simulink model "SystemModel"  (R2020b)
settings: Solver=VariableStepAuto  StartTime=0.0  StopTime=0.1  RelTol=1e-3
PostLoadFcn:
  | ModelInit
undefined symbols (not defined in the file): F_PWM
libraries: nesl_utility x25, fl_lib x24, ee_lib x22, powerlib_meascontrol x2
(part 1 of 2)
settings Model: Creator=on4ip  LastModifiedBy=on4ip
settings SolverCC: AutoInsertRateTranBlk=on
settings OptimizationCC: UseDivisionForNetSlopeComputation=on
settings ModelReferenceCC: EnableRefExpFcnMdlSchedulingChecks=off

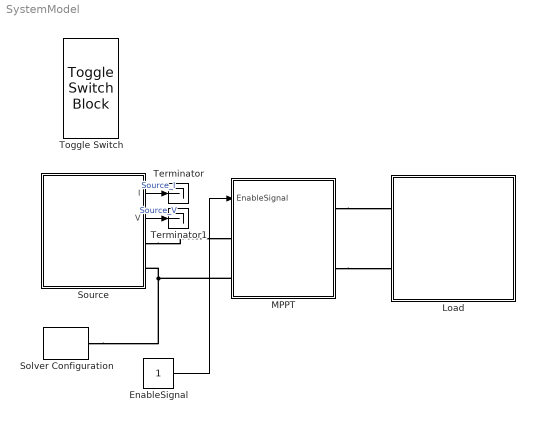
== system SystemModel ==
  EnableSignal : Constant
  Load : Subsystem
  MPPT : Subsystem
  Solver Configuration : nesl_utility/Solver Configuration  PhysicalDomain=network_engine_domain  SubClassName=solver  LeftPortType=input  RightPortType=generic  Tones=[]  Harmonics=[]  SimulateNoise=off  Profile=off  UseLocalSampling=off  EnableSwitchedLinearOptims=on  FrequencyDomain=off  UseCCode=off  RelTol=0.001  AbsTol=1e-06  MinStep=1e-09  ToWorkspace=off  RevertToSquareIcSolve=off  NumHomotopyIterations=100  PhasorMode=off  PhasorModeNumHarmonics=1  DoDC=on  ResidualTolerance=1e-09  UseLocalSolver=off  LocalSolverChoice=NE_BACKWARD_EULER_ADVANCER  LocalSolverSampleTime=1/10e6  DoFixedCost=off  MaxNonlinIter=3  MaxModeIter=2  ComputeImpulses=off  ImpulseIterations=2  LinearAlgebra=auto  EquationFormulation=NE_TIME_EF  DelaysMemoryBudget=1024  AutomaticFiltering=on  FilteringTimeConstant=0.001  PartitionStorageMethod=AS_NEEDED  PartitionMemoryBudget=1024  PartitionMethod=ROBUST
  Source : Subsystem  AncestorBlock=slexMaskingVariants_libraryblock/VariantSubsystem2  Variant=on  VariantControlMode=label  LabelModeActiveChoice=DCvariant  mask{VChoice=DC, Vnom=120}
      mask prompts: VChoice "Select a source variant"; Vnom "Nominal Voltage"
      mask init:
      | choice = get_param(gcb,'VChoice');
      | vssBlk = gcb;
      | oldVariant = get_param(gcb,'LabelModeActiveChoice');
      | if strcmp(choice,'DC')
      |     
      |     set_param(vssBlk, 'LabelModeActiveChoice', 'DCvariant');
      | else
      |     
      |     set_param(vssBlk, 'LabelModeActiveChoice', 'PVvariant');
      | end
      mask TypeOptions VChoice: DC | PV
      mask DialogControl DescGroupVar Prompt: Source Model Mask
      mask DialogControl DescTextVar Prompt: Выбор модели для источника питания
  Terminator : Terminator
  Terminator1 : Terminator
  Toggle Switch : ToggleSwitchBlock
      settings: Values={{'Off', 'On'}, [0 1]}
  wires:
  Source/1(I) -> Terminator/1  "Source_I"
  Source/2(V) -> Terminator1/1  "Source_V"
  EnableSignal/1 -> MPPT/1(EnableSignal)
  connections:
  Solver Configuration/RConn1 -- Source/RConn2 -- MPPT/LConn2
  Source/RConn1 -- MPPT/LConn1
  MPPT/RConn1 -- Load/LConn1
  MPPT/RConn2 -- Load/LConn2

== system SystemModel/Load ==
  Resistor : fl_lib/Electrical/Electrical Elements/Resistor  R=4 Ohm  i_specify=off  i_priority=None  i=0 A  i_nominal_specify=off  i_nominal_unit=A  i_nominal_value=1  v_specify=off  v_priority=None  v=0 V  v_nominal_specify=off  v_nominal_unit=V  v_nominal_value=1
  Load+ : PMIOPort  Side=Left
  Load- : PMIOPort  Port=2  Side=Left
  connections:
  Resistor/LConn1 -- Load+/RConn1
  Load-/RConn1 -- Resistor/RConn1

== system SystemModel/MPPT ==
  note: Для просмотра структуры конвертера
      | нажмите ЗДЕСЬ
  EnableSignal : Inport
  MCU : Subsystem
      settings: PortSchema="{\"entries\":[{\"content\":{\"sides\":[{\"content\":{\"connectorIds\":[\"Out1\"]},\"type\":\"ConnectorPlacement.EquallySpacedRectSide\",\"uuid\":\"95aacd01-5f53-4576-9898-5de1b84e2e57\"},{\"content\":{\"connectorIds\":[\"In1\"],\"side\":\"RIGHT\"},\"type\":\"ConnectorPlacement.EquallySpacedRectSide\",\"uuid\":\"70467306-ac55-4107-9f3e-d6d472329373\"},{\"content\":{\"connectorIds\":[],\"side\":\"TOP\"},\"type\":\"ConnectorPlacement.EquallySpacedRectSide\",\"uuid\":\"582591cf-2fae-45e2-b4f1-703e68dc17d8\"},{\"content\":{\"connectorIds\":[],\"side\":\"HIDDEN\"},\"type\":\"ConnectorPlacement.EquallySpacedRectSide\",\"uuid\":\"e5d6186a-71bc-43f6-a780-6a1a666a1cb3\"}]},\"type\":\"ConnectorPlacement.EquallySpacedConnector\",\"uuid\":\"3fd99db7-1fcf-4f0b-8db4-a60f3c66b2ee\"}],\"packageUris\":[\"http://schema.mathworks.com/mf0/Connector/R2020b\"],\"version\":\"1.0\"}"
  PhisicalModel : Subsystem
  IN+ : PMIOPort  Side=Left
  IN- : PMIOPort  Port=2  Side=Left
  Out+ : PMIOPort  Port=3  Side=Right
  Out- : PMIOPort  Port=4  Side=Right
  wires:
  MCU/1(Control_Signals) -> PhisicalModel/2(Control_Signals)
  PhisicalModel/1(Feedback_Signals) -> MCU/1(Feedback_Signals)
  EnableSignal/1 -> PhisicalModel/1(EnableSignal)
  connections:
  IN+/RConn1 -- PhisicalModel/LConn1
  IN-/RConn1 -- PhisicalModel/LConn2
  Out+/RConn1 -- PhisicalModel/RConn1
  Out-/RConn1 -- PhisicalModel/RConn2

== system SystemModel/Source ==
  note: 1) Add Subsystem or Model blocks as valid variant choices.
      | 2) You cannot connect blocks at this level. At simulation, connectivity is automatically
      | determined, based on the active variant and port name matching.
  DC source : Subsystem  VariantControl=DCvariant
  PV source : Subsystem  VariantControl=PVvariant
  + : PMIOPort  Side=Right
  - : PMIOPort  Port=2  Side=Right
  I : Outport  VectorParamsAs1DForOutWhenUnconnected=off
  V : Outport  Port=2  VectorParamsAs1DForOutWhenUnconnected=off

== system SystemModel/MPPT/MCU ==
  Feedback_Signals : Inport
  Bus Creator : BusCreator  Inputs=5
  Bus Selector : BusSelector  OutputSignals=PWM_ref,Ena,OPTO_1,OPTO_2,OPTO_3
  ControlMCU : ModelReference  ModelNameDialog=MpptControl.slx  SimulationMode=Normal  ScheduleRates=on  ModelReferenceVersion=1.23
      settings: PortSchema="{\"entries\":[{\"content\":{\"sides\":[{\"content\":{\"connectorIds\":[\"In2\",\"In1\"]},\"type\":\"ConnectorPlacement.EquallySpacedRectSide\",\"uuid\":\"62c77ea2-8a62-4ba9-937a-755ecaf63dee\"},{\"content\":{\"connectorIds\":[\"Out1\"],\"side\":\"RIGHT\"},\"type\":\"ConnectorPlacement.EquallySpacedRectSide\",\"uuid\":\"565939dd-5422-42ba-a796-bcc2d661967f\"},{\"content\":{\"connectorIds\":[],\"side\":\"TOP\"},\"type\":\"ConnectorPlacement.EquallySpacedRectSide\",\"uuid\":\"40f1e559-ba9a-42bc-8a75-57ac09117705\"},{\"content\":{\"connectorIds\":[],\"side\":\"HIDDEN\"},\"type\":\"ConnectorPlacement.EquallySpacedRectSide\",\"uuid\":\"e8af7b68-8515-405e-bf62-830d8685ff5a\"}]},\"type\":\"ConnectorPlacement.EquallySpacedConnector\",\"uuid\":\"8beb7fe5-f4a1-4e5e-a07e-3689976499a8\"}],\"packageUris\":[\"http://schema.mathworks.com/mf0/Connector/R2020b\"],\"version\":\"1.0\"}"
  MCU PWM : Subsystem  mask{Fpwm=F_PWM}
      mask prompts: Fpwm "PWM frequency"
  SignalPack : Subsystem
  Unit Delay : UnitDelay  SampleTime=-1  HasFrameUpgradeWarning=on
  Control_Signals : Outport
  wires:
  Bus Creator/1 -> Control_Signals/1
  Feedback_Signals/1 -> SignalPack/1(In1)
  MCU PWM/3(INB) -> Bus Creator/2  "INB"
  MCU PWM/2(INA) -> Bus Creator/1  "INA"
  Bus Selector/2 -> MCU PWM/2(Ena)  "<Ena>"
  Bus Selector/3 -> Bus Creator/3  "<OPTO_1>"
  Bus Selector/4 -> Bus Creator/4  "<OPTO_2>"
  Bus Selector/5 -> Bus Creator/5  "<OPTO_3>"
  ControlMCU/1 -> Unit Delay/1
  Unit Delay/1 -> Bus Selector/1
  SignalPack/1(FeedBack) -> ControlMCU/1
  Bus Selector/1 -> MCU PWM/1(Ref)  "<PWM_ref>"
  MCU PWM/1(ISR) -> ControlMCU/2

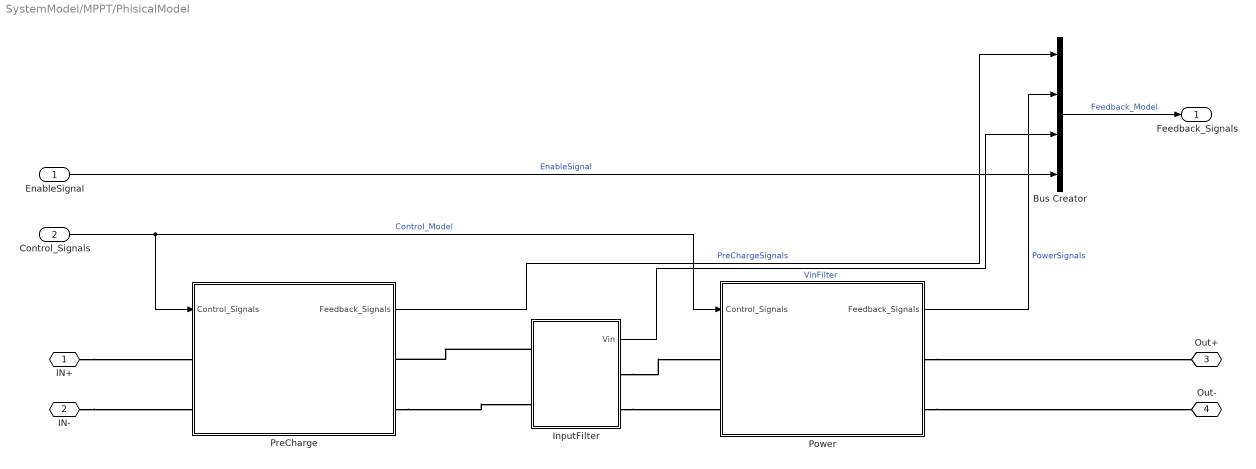
== system SystemModel/MPPT/PhisicalModel ==
  EnableSignal : Inport
  Control_Signals : Inport  Port=2
  Bus Creator : BusCreator  Inputs=4
  InputFilter : Subsystem  mask{Lf=20, Cf=11}
      mask prompts: Lf "Input filter Inductance,uH"; Cf "Input filter Capacitance,uF"
  Power : Subsystem  mask{Ls=200, Rs=30e-3, Cout=1000, Cf=2200, Lf=100}
      mask prompts: Ls "Inductor value,uH"; Rs "Inductor Resistance,Omh"; Cout "Out capacitor value,uF"; Cf "Filter capacitor value,uF"; Lf "Filter inductance value,uH"
  PreCharge : Subsystem
  IN+ : PMIOPort  Side=Left
  IN- : PMIOPort  Port=2  Side=Left
  Out+ : PMIOPort  Port=3  Side=Right
  Out- : PMIOPort  Port=4  Side=Right
  Feedback_Signals : Outport
  wires:
  Control_Signals/1 -> PreCharge/1(Control_Signals), Power/1(Control_Signals)  "Control_Model"
  Power/1(Feedback_Signals) -> Bus Creator/2  "PowerSignals"
  PreCharge/1(Feedback_Signals) -> Bus Creator/1  "PreChargeSignals"
  Bus Creator/1 -> Feedback_Signals/1  "Feedback_Model"
  InputFilter/1(Vin) -> Bus Creator/3  "VinFilter"
  EnableSignal/1 -> Bus Creator/4  "EnableSignal"
  connections:
  IN+/RConn1 -- PreCharge/LConn1
  IN-/RConn1 -- PreCharge/LConn2
  Power/RConn1 -- Out+/RConn1
  Power/RConn2 -- Out-/RConn1
  InputFilter/LConn1 -- PreCharge/RConn1
  PreCharge/RConn2 -- InputFilter/LConn2
  InputFilter/RConn1 -- Power/LConn1
  InputFilter/RConn2 -- Power/LConn2

== system SystemModel/Source/DC source ==
  Electrical Reference : fl_lib/Electrical/Electrical Elements/Electrical Reference
  Sensors : Subsystem
  Voltage Source : ee_lib/Sources/Voltage Source  dc_voltage=Vnom V  ac_voltage=0 V  ac_shift=0 rad  ac_frequency=60 Hz  noise_mode=0  PSD=0 V^2/Hz  repeatability=1  auto_seed=1503168829  user_seed=0  sample_time=1e-3 s  i_specify=off  i_priority=None  i=0 A  i_nominal_specify=off  i_nominal_unit=A  i_nominal_value=1  v_specify=off  v_priority=None  v=0 V  v_nominal_specify=off  v_nominal_unit=V  v_nominal_value=1
  + : PMIOPort  Side=Right
  - : PMIOPort  Port=2  Side=Right
  I : Outport  VectorParamsAs1DForOutWhenUnconnected=off
  V : Outport  Port=2  VectorParamsAs1DForOutWhenUnconnected=off
  wires:
  Sensors/1(I) -> I/1
  Sensors/2(V) -> V/1
  connections:
  Sensors/LConn1 -- Voltage Source/LConn1
  Voltage Source/RConn1 -- Electrical Reference/LConn1 -- Sensors/LConn2
  Sensors/RConn1 -- +/RConn1
  -/RConn1 -- Sensors/RConn2

== system SystemModel/Source/PV source ==
  Electrical Reference : fl_lib/Electrical/Electrical Elements/Electrical Reference
  Sensors : Subsystem
  Voltage Source : ee_lib/Sources/Voltage Source  dc_voltage=0 V  ac_voltage=0 V  ac_shift=0 rad  ac_frequency=60 Hz  noise_mode=0  PSD=0 V^2/Hz  repeatability=1  auto_seed=1582629291  user_seed=0  sample_time=1e-3 s  i_specify=off  i_priority=None  i=0 A  i_nominal_specify=off  i_nominal_unit=A  i_nominal_value=1  v_specify=off  v_priority=None  v=0 V  v_nominal_specify=off  v_nominal_unit=V  v_nominal_value=1
  + : PMIOPort  Side=Right
  - : PMIOPort  Port=2  Side=Right
  I : Outport  VectorParamsAs1DForOutWhenUnconnected=off
  V : Outport  Port=2  VectorParamsAs1DForOutWhenUnconnected=off
  wires:
  Sensors/1(I) -> I/1
  Sensors/2(V) -> V/1
  connections:
  Sensors/RConn1 -- +/RConn1
  Sensors/LConn1 -- Voltage Source/LConn1
  -/RConn1 -- Sensors/RConn2
  Voltage Source/RConn1 -- Electrical Reference/LConn1 -- Sensors/LConn2

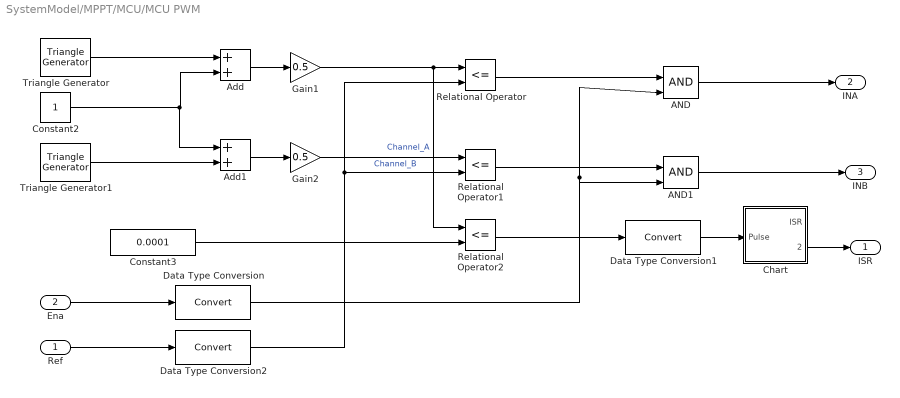
== system SystemModel/MPPT/MCU/MCU PWM ==
  Ref : Inport
  Ena : Inport  Port=2
  AND : Logic  IconShape=distinctive  AllPortsSameDT=off  OutDataTypeStr=boolean
  AND1 : Logic  IconShape=distinctive  AllPortsSameDT=off  OutDataTypeStr=boolean
  Add : Sum
  Add1 : Sum
  Chart : Stateflow chart  TreatAsAtomicUnit=on
  Constant2 : Constant
  Constant3 : Constant  Value=0.0001
  Data Type Conversion : DataTypeConversion
  Data Type Conversion1 : DataTypeConversion
  Data Type Conversion2 : DataTypeConversion
  Gain1 : Gain  Gain=0.5
  Gain2 : Gain  Gain=0.5
  Relational Operator : RelationalOperator  Operator=<=  OutDataTypeStr=boolean  ZeroCross=off  RndMeth=Simplest
  Relational Operator1 : RelationalOperator  Operator=<=  OutDataTypeStr=boolean  ZeroCross=off  RndMeth=Simplest
  Relational Operator2 : RelationalOperator  Operator=<=  OutDataTypeStr=boolean  RndMeth=Simplest
  Triangle Generator : powerlib_meascontrol/Pulse & Signal Generators/Triangle Generator  Freq=Fpwm  Phase=0  Ts=1/(Fpwm*100)
  Triangle Generator1 : powerlib_meascontrol/Pulse & Signal Generators/Triangle Generator  Freq=Fpwm  Phase=180  Ts=1/(Fpwm*100)
  ISR : Outport
  INA : Outport  Port=2
  INB : Outport  Port=3
  wires:
  Add/1 -> Gain1/1
  Relational Operator/1 -> AND/1
  Relational Operator1/1 -> AND1/1
  Ena/1 -> Data Type Conversion/1
  Ref/1 -> Data Type Conversion2/1
  Add1/1 -> Gain2/1
  Triangle Generator/1 -> Add/1
  Constant2/1 -> Add1/1, Add/2
  Triangle Generator1/1 -> Add1/2
  Gain1/1 -> Relational Operator2/1, Relational Operator/1  "Channel_A"
  Gain2/1 -> Relational Operator1/1  "Channel_B"
  Relational Operator2/1 -> Data Type Conversion1/1
  Constant3/1 -> Relational Operator2/2
  Data Type Conversion/1 -> AND/2, AND1/2
  Data Type Conversion2/1 -> Relational Operator/2, Relational Operator1/2
  AND/1 -> INA/1
  AND1/1 -> INB/1
  Data Type Conversion1/1 -> Chart/1(Pulse)
  Chart/2(ISR_event()) -> ISR/1

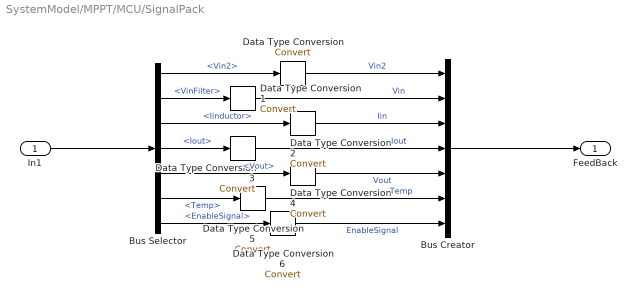
== system SystemModel/MPPT/MCU/SignalPack ==
  In1 : Inport
  Bus Creator : BusCreator  Inputs=7
  Bus Selector : BusSelector  OutputSignals=PreChargeSignals.Vin2,VinFilter,PowerSignals.Iinductor,PowerSignals.Iout,PowerSignals.Vout,PowerSignals.Temp,EnableSignal
  Data Type Conversion{,1..6} (7 alike) : DataTypeConversion
  FeedBack : Outport
  wires:
  Bus Selector/1 -> Data Type Conversion/1  "<Vin2>"
  Bus Selector/3 -> Data Type Conversion2/1  "<Iinductor>"
  Bus Selector/4 -> Data Type Conversion3/1  "<Iout>"
  Bus Selector/5 -> Data Type Conversion4/1  "<Vout>"
  Bus Selector/6 -> Data Type Conversion5/1  "<Temp>"
  Data Type Conversion/1 -> Bus Creator/1  "Vin2"
  Data Type Conversion1/1 -> Bus Creator/2  "Vin"
  Data Type Conversion2/1 -> Bus Creator/3  "Iin"
  Data Type Conversion3/1 -> Bus Creator/4  "Iout"
  Data Type Conversion4/1 -> Bus Creator/5  "Vout"
  Data Type Conversion5/1 -> Bus Creator/6  "Temp"
  In1/1 -> Bus Selector/1
  Bus Creator/1 -> FeedBack/1
  Bus Selector/2 -> Data Type Conversion1/1  "<VinFilter>"
  Bus Selector/7 -> Data Type Conversion6/1  "<EnableSignal>"
  Data Type Conversion6/1 -> Bus Creator/7  "EnableSignal"

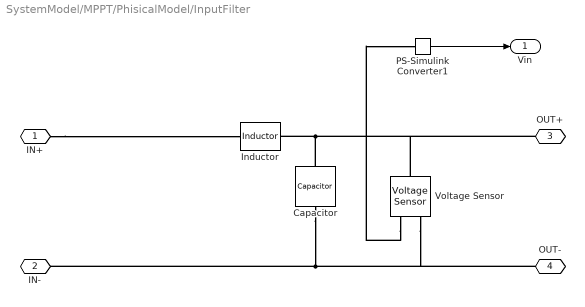
== system SystemModel/MPPT/PhisicalModel/InputFilter ==
  Capacitor : fl_lib/Electrical/Electrical Elements/Capacitor  c=Cf uF  r=1e-6 Ohm  g=0 1/Ohm  i_specify=off  i_priority=None  i=0 A  i_nominal_specify=off  i_nominal_unit=A  i_nominal_value=1  v_specify=off  v_priority=None  v=0 V  v_nominal_specify=off  v_nominal_unit=V  v_nominal_value=1  vc_specify=off  vc_priority=High  vc=0 V  vc_nominal_specify=off  vc_nominal_unit=V  vc_nominal_value=1
  Inductor : ee_lib/Passive/Inductor  l=Lf uH  L_tol=20  enable_L_tol=0  tol_distribution=1  nSigma=4  r=1e-3 Ohm  g=1e-9 1/Ohm  enable_operating_limits=0  operating_limit_action=2  max_working_current=1 A  power_rating=1 W  enable_faults=0  fault_action=1  lambdaPercent=50  k_faulted=0.9999  turnsShort=0  openCct=0  groundShort=0  groundShortG=0 1/Ohm  tau_fault=1e-3 s  enable_temporal_fault=0  t_fault=1 s  enable_behavioral_fault=0  max_permissible_voltage=100 V  n_fail_on_voltage=1  max_permissible_current=1 A  t_fail_on_current=1 s  i_L_specify=off  i_L_priority=High  i_L=0 A  i_L_nominal_specify=off  i_L_nominal_unit=A  i_L_nominal_value=1
  PS-Simulink Converter1 : nesl_utility/PS-Simulink Converter  PhysicalDomain=network_engine_domain  SubClassName=ps_output  LeftPortType=input  RightPortType=output  PseudoPeriodic=off  Frequencies=[]  Unit=inherit  AffineConversion=off
  Voltage Sensor : fl_lib/Electrical/Electrical Sensors/Voltage Sensor
  IN+ : PMIOPort  Side=Left
  IN- : PMIOPort  Port=2  Side=Left
  OUT+ : PMIOPort  Port=3  Side=Right
  OUT- : PMIOPort  Port=4  Side=Right
  Vin : Outport
  wires:
  PS-Simulink Converter1/1 -> Vin/1
  connections:
  IN+/RConn1 -- Inductor/LConn1
  Capacitor/LConn1 -- Voltage Sensor/LConn1 -- OUT+/RConn1 -- Inductor/RConn1
  Capacitor/RConn1 -- Voltage Sensor/RConn2 -- OUT-/RConn1 -- IN-/RConn1
  Voltage Sensor/RConn1 -- PS-Simulink Converter1/LConn1

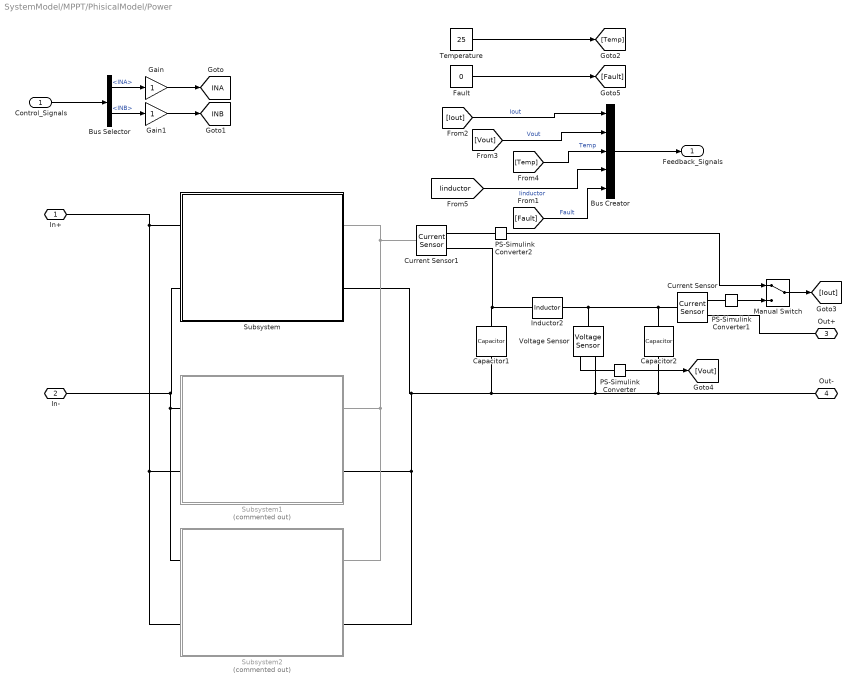
== system SystemModel/MPPT/PhisicalModel/Power ==
  Control_Signals : Inport
  Bus Creator : BusCreator  Inputs=5
  Bus Selector : BusSelector  OutputSignals=INA,INB
  Capacitor1 : fl_lib/Electrical/Electrical Elements/Capacitor  c=Cout uF  r=1e-6 Ohm  g=0 1/Ohm  i_specify=off  i_priority=None  i=0 A  i_nominal_specify=off  i_nominal_unit=A  i_nominal_value=1  v_specify=off  v_priority=None  v=0 V  v_nominal_specify=off  v_nominal_unit=V  v_nominal_value=1  vc_specify=off  vc_priority=High  vc=0 V  vc_nominal_specify=off  vc_nominal_unit=V  vc_nominal_value=1
  Capacitor2 : fl_lib/Electrical/Electrical Elements/Capacitor  c=Cf uF  r=1e-6 Ohm  g=0 1/Ohm  i_specify=off  i_priority=None  i=0 A  i_nominal_specify=off  i_nominal_unit=A  i_nominal_value=1  v_specify=off  v_priority=None  v=0 V  v_nominal_specify=off  v_nominal_unit=V  v_nominal_value=1  vc_specify=off  vc_priority=High  vc=0 V  vc_nominal_specify=off  vc_nominal_unit=V  vc_nominal_value=1
  Current Sensor : fl_lib/Electrical/Electrical Sensors/Current Sensor
  Current Sensor1 : fl_lib/Electrical/Electrical Sensors/Current Sensor
  Fault : Constant  Value=0  OutDataTypeStr=Inherit: Inherit via back propagation
  Gain : Gain  OutDataTypeStr=double
  Gain1 : Gain  OutDataTypeStr=double
  Inductor2 : ee_lib/Passive/Inductor  l=Lf nH  L_tol=20  enable_L_tol=0  tol_distribution=1  nSigma=4  r=0 Ohm  g=1e-9 1/Ohm  enable_operating_limits=0  operating_limit_action=2  max_working_current=1 A  power_rating=1 W  enable_faults=0  fault_action=1  lambdaPercent=50  k_faulted=0.9999  turnsShort=0  openCct=0  groundShort=0  groundShortG=0 1/Ohm  tau_fault=1e-3 s  enable_temporal_fault=0  t_fault=1 s  enable_behavioral_fault=0  max_permissible_voltage=100 V  n_fail_on_voltage=1  max_permissible_current=1 A  t_fail_on_current=1 s  i_L_specify=off  i_L_priority=High  i_L=0 A  i_L_nominal_specify=off  i_L_nominal_unit=A  i_L_nominal_value=1
  Manual Switch : ManualSwitch
  PS-Simulink Converter : nesl_utility/PS-Simulink Converter  PhysicalDomain=network_engine_domain  SubClassName=ps_output  LeftPortType=input  RightPortType=output  PseudoPeriodic=off  Frequencies=[]  Unit=inherit  AffineConversion=off
  PS-Simulink Converter1 : nesl_utility/PS-Simulink Converter  PhysicalDomain=network_engine_domain  SubClassName=ps_output  LeftPortType=input  RightPortType=output  PseudoPeriodic=off  Frequencies=[]  Unit=inherit  AffineConversion=off
  PS-Simulink Converter2 : nesl_utility/PS-Simulink Converter  PhysicalDomain=network_engine_domain  SubClassName=ps_output  LeftPortType=input  RightPortType=output  PseudoPeriodic=off  Frequencies=[]  Unit=inherit  AffineConversion=off
  Subsystem : Subsystem
  Subsystem1 : Subsystem  Commented=on
  Subsystem2 : Subsystem  Commented=on
  Temperature : Constant  Value=25  OutDataTypeStr=Inherit: Inherit via back propagation
  Voltage Sensor : fl_lib/Electrical/Electrical Sensors/Voltage Sensor
  In+ : PMIOPort  Side=Left
  In- : PMIOPort  Port=2  Side=Left
  Out+ : PMIOPort  Port=3  Side=Right
  Out- : PMIOPort  Port=4  Side=Right
  Feedback_Signals : Outport
  tag scope: INA=global, INB=global
  wires:
  Control_Signals/1 -> Bus Selector/1
  Bus Selector/1 -> Gain/1  "<INA>"
  Bus Selector/2 -> Gain1/1  "<INB>"
  Temperature/1 -> [Temp]
  PS-Simulink Converter/1 -> [Vout]
  Bus Creator/1 -> Feedback_Signals/1
  [Iout] -> Bus Creator/1  "Iout"
  [Temp] -> Bus Creator/3  "Temp"
  [Vout] -> Bus Creator/2  "Vout"
  Gain/1 -> [INA]
  Gain1/1 -> [INB]
  [Iinductor] -> Bus Creator/4  "Iinductor"
  PS-Simulink Converter2/1 -> Manual Switch/1
  PS-Simulink Converter1/1 -> Manual Switch/2
  Manual Switch/1 -> [Iout]
  Fault/1 -> [Fault]
  [Fault] -> Bus Creator/5  "Fault"
  connections:
  Subsystem/LConn2 -- Subsystem2/LConn1 -- Subsystem1/LConn1 -- In-/RConn1
  Inductor2/LConn1 -- Current Sensor1/RConn2 -- Capacitor1/LConn1
  Out+/RConn1 -- Current Sensor/RConn2
  Capacitor2/LConn1 -- Voltage Sensor/LConn1 -- Inductor2/RConn1 -- Current Sensor/LConn1
  PS-Simulink Converter/LConn1 -- Voltage Sensor/RConn1
  PS-Simulink Converter1/LConn1 -- Current Sensor/RConn1
  Subsystem/LConn1 -- Subsystem2/LConn2 -- Subsystem1/LConn2 -- In+/RConn1
  Voltage Sensor/RConn2 -- Subsystem2/RConn2 -- Subsystem1/RConn2 -- Subsystem/RConn2 -- Capacitor1/RConn1 -- Out-/RConn1 -- Capacitor2/RConn1
  Subsystem1/RConn1 -- Current Sensor1/LConn1 -- Subsystem/RConn1 -- Subsystem2/RConn1
  PS-Simulink Converter2/LConn1 -- Current Sensor1/RConn1

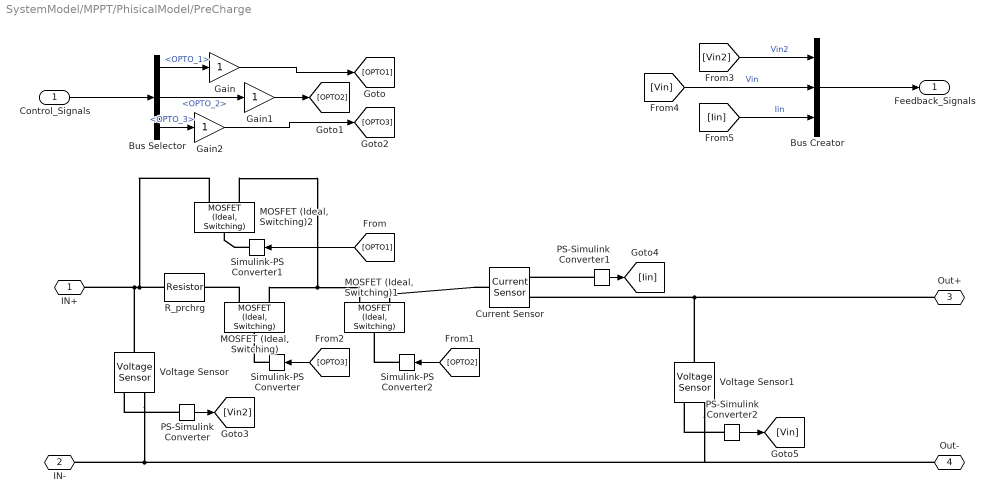
== system SystemModel/MPPT/PhisicalModel/PreCharge ==
  Control_Signals : Inport
  Bus Creator : BusCreator  Inputs=3
  Bus Selector : BusSelector  OutputSignals=OPTO_1,OPTO_2,OPTO_3
  Current Sensor : fl_lib/Electrical/Electrical Sensors/Current Sensor
  Gain : Gain  OutDataTypeStr=double
  Gain1 : Gain  OutDataTypeStr=double
  Gain2 : Gain  OutDataTypeStr=double
  "MOSFET (Ideal, Switching)" : ee_lib/Semiconductors & Converters/MOSFET (Ideal, Switching)  Rds=56e-3 Ohm  Goff=1e-6 1/Ohm  Vth=0.5 V  diode_param=2  diode_Vf=0.8 V  diode_Ron=0.001 Ohm  diode_Goff=1e-5 1/Ohm  diode_C=50e-9 F  diode_iRM=-235 A  diode_iF=300 A  diode_idot=-50 A/us  diode_trr_param=1  diode_trr_factor=3  diode_trr=15 us  diode_Qrr=1500 s*uA  thermal_loss_option=ee.enum.converters.thermalLossOption.constantvalues  Von_data=[0, 1.1, 1.3, 1.45, 1.75, 2.25, 2.7; 0, 1, 1.15, 1.35, 1.7, 2.35, 3] V  Eon_data=[0, .29, 1.43, 2.86, 5.71, 13.14, 22.86; 0, .57, 2.63, 5.14, 10.29, 20.57, 30.29] * 1e-3 J  Eoff_data=[0, .21, 1.07, 2.14, 4.29, 9.86, 17.14; 0, .43, 1.97, 3.86, 7.71, 15.43, 22.71] * 1e-3 J  Tj=[298.15, 398.15] K  Iout_data=[0, 10, 50, 100, 200, 400, 600] A  Eon_scalar=22.86e-3 J  Eoff_scalar=17.14e-3 J  Voff=300 V  Iout_scalar=600 A  diodeModelType=ee.enum.converters.diodeModelType.pwl  diode_IfMat=[.07, .12, .19, 1.75, 4.24, 7.32, 11.2; .16, .3, .72, 2.14, 4.02, 6.35, 9.12] A  diode_TjVec=[25, 125] degC  diode_VfVec=[.5, .7, .9, 1.3, 1.7, 2.1, 2.5] V  thermal_network_parameterization=ee.enum.thermalNetworkTopology.external  Rth=[.03, .2] K/W  Rth_Foster=[.03, .2] K/W  thermal_mass_parameterization=ee.enum.thermalNetwork.timeconstant  thermal_mass=[3, 25] J/K  thermal_mass_Foster=[33, 50] J/K  thermal_time_constant=[.1, 5] s  thermal_time_constant_Foster=[1, 10] s  thermal_mass_initial_temperatures=[25, 25] degC  junction_thermal_mass=0.1 J/K  Tau=1e-4 s  vT_specify=off  vT_priority=None  vT=0 V  vT_nominal_specify=off  vT_nominal_unit=V  vT_nominal_value=1  Qj_specify=off  Qj_priority=None  Qj=0 W  Qj_nominal_specify=off  Qj_nominal_unit=W  Qj_nominal_value=1  junction_temperature_specify=off  junction_temperature_priority=None  junction_temperature=25 degC  junction_temperature_nominal_specify=off  junction_temperature_nominal_unit=degC  junction_temperature_nominal_value=1
  "MOSFET (Ideal, Switching)1" : ee_lib/Semiconductors & Converters/MOSFET (Ideal, Switching)  Rds=56e-3 Ohm  Goff=1e-6 1/Ohm  Vth=0.5 V  diode_param=2  diode_Vf=0.8 V  diode_Ron=0.001 Ohm  diode_Goff=1e-5 1/Ohm  diode_C=50e-9 F  diode_iRM=-235 A  diode_iF=300 A  diode_idot=-50 A/us  diode_trr_param=1  diode_trr_factor=3  diode_trr=15 us  diode_Qrr=1500 s*uA  thermal_loss_option=ee.enum.converters.thermalLossOption.constantvalues  Von_data=[0, 1.1, 1.3, 1.45, 1.75, 2.25, 2.7; 0, 1, 1.15, 1.35, 1.7, 2.35, 3] V  Eon_data=[0, .29, 1.43, 2.86, 5.71, 13.14, 22.86; 0, .57, 2.63, 5.14, 10.29, 20.57, 30.29] * 1e-3 J  Eoff_data=[0, .21, 1.07, 2.14, 4.29, 9.86, 17.14; 0, .43, 1.97, 3.86, 7.71, 15.43, 22.71] * 1e-3 J  Tj=[298.15, 398.15] K  Iout_data=[0, 10, 50, 100, 200, 400, 600] A  Eon_scalar=22.86e-3 J  Eoff_scalar=17.14e-3 J  Voff=300 V  Iout_scalar=600 A  diodeModelType=ee.enum.converters.diodeModelType.pwl  diode_IfMat=[.07, .12, .19, 1.75, 4.24, 7.32, 11.2; .16, .3, .72, 2.14, 4.02, 6.35, 9.12] A  diode_TjVec=[25, 125] degC  diode_VfVec=[.5, .7, .9, 1.3, 1.7, 2.1, 2.5] V  thermal_network_parameterization=ee.enum.thermalNetworkTopology.external  Rth=[.03, .2] K/W  Rth_Foster=[.03, .2] K/W  thermal_mass_parameterization=ee.enum.thermalNetwork.timeconstant  thermal_mass=[3, 25] J/K  thermal_mass_Foster=[33, 50] J/K  thermal_time_constant=[.1, 5] s  thermal_time_constant_Foster=[1, 10] s  thermal_mass_initial_temperatures=[25, 25] degC  junction_thermal_mass=0.1 J/K  Tau=1e-4 s  vT_specify=off  vT_priority=None  vT=0 V  vT_nominal_specify=off  vT_nominal_unit=V  vT_nominal_value=1  Qj_specify=off  Qj_priority=None  Qj=0 W  Qj_nominal_specify=off  Qj_nominal_unit=W  Qj_nominal_value=1  junction_temperature_specify=off  junction_temperature_priority=None  junction_temperature=25 degC  junction_temperature_nominal_specify=off  junction_temperature_nominal_unit=degC  junction_temperature_nominal_value=1
  "MOSFET (Ideal, Switching)2" : ee_lib/Semiconductors & Converters/MOSFET (Ideal, Switching)  Rds=56e-3 Ohm  Goff=1e-6 1/Ohm  Vth=0.5 V  diode_param=2  diode_Vf=0.8 V  diode_Ron=0.001 Ohm  diode_Goff=1e-5 1/Ohm  diode_C=50e-9 F  diode_iRM=-235 A  diode_iF=300 A  diode_idot=-50 A/us  diode_trr_param=1  diode_trr_factor=3  diode_trr=15 us  diode_Qrr=1500 s*uA  thermal_loss_option=ee.enum.converters.thermalLossOption.constantvalues  Von_data=[0, 1.1, 1.3, 1.45, 1.75, 2.25, 2.7; 0, 1, 1.15, 1.35, 1.7, 2.35, 3] V  Eon_data=[0, .29, 1.43, 2.86, 5.71, 13.14, 22.86; 0, .57, 2.63, 5.14, 10.29, 20.57, 30.29] * 1e-3 J  Eoff_data=[0, .21, 1.07, 2.14, 4.29, 9.86, 17.14; 0, .43, 1.97, 3.86, 7.71, 15.43, 22.71] * 1e-3 J  Tj=[298.15, 398.15] K  Iout_data=[0, 10, 50, 100, 200, 400, 600] A  Eon_scalar=22.86e-3 J  Eoff_scalar=17.14e-3 J  Voff=300 V  Iout_scalar=600 A  diodeModelType=ee.enum.converters.diodeModelType.pwl  diode_IfMat=[.07, .12, .19, 1.75, 4.24, 7.32, 11.2; .16, .3, .72, 2.14, 4.02, 6.35, 9.12] A  diode_TjVec=[25, 125] degC  diode_VfVec=[.5, .7, .9, 1.3, 1.7, 2.1, 2.5] V  thermal_network_parameterization=ee.enum.thermalNetworkTopology.external  Rth=[.03, .2] K/W  Rth_Foster=[.03, .2] K/W  thermal_mass_parameterization=ee.enum.thermalNetwork.timeconstant  thermal_mass=[3, 25] J/K  thermal_mass_Foster=[33, 50] J/K  thermal_time_constant=[.1, 5] s  thermal_time_constant_Foster=[1, 10] s  thermal_mass_initial_temperatures=[25, 25] degC  junction_thermal_mass=0.1 J/K  Tau=1e-4 s  vT_specify=off  vT_priority=None  vT=0 V  vT_nominal_specify=off  vT_nominal_unit=V  vT_nominal_value=1  Qj_specify=off  Qj_priority=None  Qj=0 W  Qj_nominal_specify=off  Qj_nominal_unit=W  Qj_nominal_value=1  junction_temperature_specify=off  junction_temperature_priority=None  junction_temperature=25 degC  junction_temperature_nominal_specify=off  junction_temperature_nominal_unit=degC  junction_temperature_nominal_value=1
  PS-Simulink Converter : nesl_utility/PS-Simulink Converter  PhysicalDomain=network_engine_domain  SubClassName=ps_output  LeftPortType=input  RightPortType=output  PseudoPeriodic=off  Frequencies=[]  Unit=inherit  AffineConversion=off
  PS-Simulink Converter1 : nesl_utility/PS-Simulink Converter  PhysicalDomain=network_engine_domain  SubClassName=ps_output  LeftPortType=input  RightPortType=output  PseudoPeriodic=off  Frequencies=[]  Unit=inherit  AffineConversion=off
  PS-Simulink Converter2 : nesl_utility/PS-Simulink Converter  PhysicalDomain=network_engine_domain  SubClassName=ps_output  LeftPortType=input  RightPortType=output  PseudoPeriodic=off  Frequencies=[]  Unit=inherit  AffineConversion=off
  R_prchrg : fl_lib/Electrical/Electrical Elements/Resistor  R=100 Ohm  i_specify=off  i_priority=None  i=0 A  i_nominal_specify=off  i_nominal_unit=A  i_nominal_value=1  v_specify=off  v_priority=None  v=0 V  v_nominal_specify=off  v_nominal_unit=V  v_nominal_value=1
  Simulink-PS Converter : nesl_utility/Simulink-PS Converter  PhysicalDomain=network_engine_domain  SubClassName=ps_input  LeftPortType=input  RightPortType=output  PseudoPeriodic=off  Frequencies=[]  NoiseDistribution=none  NoiseParameters=[]  Unit=1  AffineConversion=off  FilteringAndDerivatives=provide  SimscapeFilterOrder=1  InputFilterTimeConstant=0.001  UdotUserProvided=0
  Simulink-PS Converter1 : nesl_utility/Simulink-PS Converter  PhysicalDomain=network_engine_domain  SubClassName=ps_input  LeftPortType=input  RightPortType=output  PseudoPeriodic=off  Frequencies=[]  NoiseDistribution=none  NoiseParameters=[]  Unit=1  AffineConversion=off  FilteringAndDerivatives=provide  SimscapeFilterOrder=1  InputFilterTimeConstant=0.001  UdotUserProvided=0
  Simulink-PS Converter2 : nesl_utility/Simulink-PS Converter  PhysicalDomain=network_engine_domain  SubClassName=ps_input  LeftPortType=input  RightPortType=output  PseudoPeriodic=off  Frequencies=[]  NoiseDistribution=none  NoiseParameters=[]  Unit=1  AffineConversion=off  FilteringAndDerivatives=provide  SimscapeFilterOrder=1  InputFilterTimeConstant=0.001  UdotUserProvided=0
  Voltage Sensor : fl_lib/Electrical/Electrical Sensors/Voltage Sensor
  Voltage Sensor1 : fl_lib/Electrical/Electrical Sensors/Voltage Sensor
  IN+ : PMIOPort  Side=Left
  IN- : PMIOPort  Port=2  Side=Left
  Out+ : PMIOPort  Port=3  Side=Right
  Out- : PMIOPort  Port=4  Side=Right
  Feedback_Signals : Outport
  wires:
  PS-Simulink Converter1/1 -> [Iin]
  Control_Signals/1 -> Bus Selector/1
  Bus Selector/1 -> Gain/1  "<OPTO_1>"
  Bus Selector/2 -> Gain1/1  "<OPTO_2>"
  Bus Selector/3 -> Gain2/1  "<OPTO_3>"
  [OPTO1] -> Simulink-PS Converter1/1
  [OPTO2] -> Simulink-PS Converter2/1
  [OPTO3] -> Simulink-PS Converter/1
  PS-Simulink Converter/1 -> [Vin2]
  PS-Simulink Converter2/1 -> [Vin]
  Bus Creator/1 -> Feedback_Signals/1
  [Vin2] -> Bus Creator/1  "Vin2"
  [Vin] -> Bus Creator/2  "Vin"
  [Iin] -> Bus Creator/3  "Iin"
  Gain/1 -> [OPTO1]
  Gain1/1 -> [OPTO2]
  Gain2/1 -> [OPTO3]
  connections:
  "MOSFET (Ideal, Switching)"/RConn2 -- "MOSFET (Ideal, Switching)2"/RConn2 -- "MOSFET (Ideal, Switching)1"/RConn2
  "MOSFET (Ideal, Switching)2"/RConn1 -- R_prchrg/LConn1 -- Voltage Sensor/LConn1 -- IN+/RConn1
  "MOSFET (Ideal, Switching)"/RConn1 -- R_prchrg/RConn1
  Voltage Sensor/RConn2 -- Out-/RConn1 -- Voltage Sensor1/RConn2 -- IN-/RConn1
  Current Sensor/LConn1 -- "MOSFET (Ideal, Switching)1"/RConn1
  Voltage Sensor1/LConn1 -- Out+/RConn1 -- Current Sensor/RConn2
  Simulink-PS Converter/RConn1 -- "MOSFET (Ideal, Switching)"/LConn1
  Simulink-PS Converter1/RConn1 -- "MOSFET (Ideal, Switching)2"/LConn1
  Simulink-PS Converter2/RConn1 -- "MOSFET (Ideal, Switching)1"/LConn1
  PS-Simulink Converter/LConn1 -- Voltage Sensor/RConn1
  PS-Simulink Converter1/LConn1 -- Current Sensor/RConn1
  PS-Simulink Converter2/LConn1 -- Voltage Sensor1/RConn1

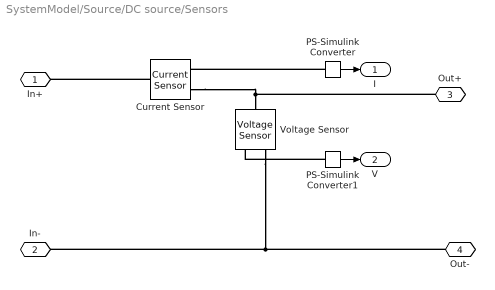
== system SystemModel/Source/DC source/Sensors ==
  Current Sensor : fl_lib/Electrical/Electrical Sensors/Current Sensor
  PS-Simulink Converter : nesl_utility/PS-Simulink Converter  PhysicalDomain=network_engine_domain  SubClassName=ps_output  LeftPortType=input  RightPortType=output  PseudoPeriodic=off  Frequencies=[]  Unit=inherit  AffineConversion=off
  PS-Simulink Converter1 : nesl_utility/PS-Simulink Converter  PhysicalDomain=network_engine_domain  SubClassName=ps_output  LeftPortType=input  RightPortType=output  PseudoPeriodic=off  Frequencies=[]  Unit=inherit  AffineConversion=off
  Voltage Sensor : fl_lib/Electrical/Electrical Sensors/Voltage Sensor
  In+ : PMIOPort  Side=Left
  In- : PMIOPort  Port=2  Side=Left
  Out+ : PMIOPort  Port=3  Side=Right
  Out- : PMIOPort  Port=4  Side=Right
  I : Outport
  V : Outport  Port=2
  wires:
  PS-Simulink Converter/1 -> I/1
  PS-Simulink Converter1/1 -> V/1
  connections:
  Current Sensor/RConn2 -- Out+/RConn1 -- Voltage Sensor/LConn1
  PS-Simulink Converter/LConn1 -- Current Sensor/RConn1
  Current Sensor/LConn1 -- In+/RConn1
  PS-Simulink Converter1/LConn1 -- Voltage Sensor/RConn1
  Out-/RConn1 -- In-/RConn1 -- Voltage Sensor/RConn2

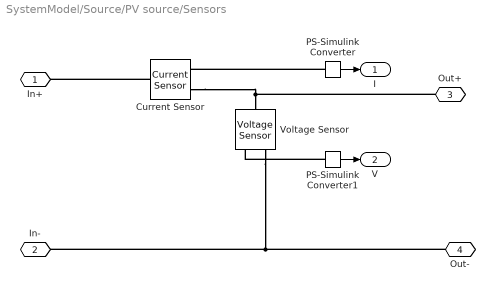
== system SystemModel/Source/PV source/Sensors ==
  Current Sensor : fl_lib/Electrical/Electrical Sensors/Current Sensor
  PS-Simulink Converter : nesl_utility/PS-Simulink Converter  PhysicalDomain=network_engine_domain  SubClassName=ps_output  LeftPortType=input  RightPortType=output  PseudoPeriodic=off  Frequencies=[]  Unit=inherit  AffineConversion=off
  PS-Simulink Converter1 : nesl_utility/PS-Simulink Converter  PhysicalDomain=network_engine_domain  SubClassName=ps_output  LeftPortType=input  RightPortType=output  PseudoPeriodic=off  Frequencies=[]  Unit=inherit  AffineConversion=off
  Voltage Sensor : fl_lib/Electrical/Electrical Sensors/Voltage Sensor
  In+ : PMIOPort  Side=Left
  In- : PMIOPort  Port=2  Side=Left
  Out+ : PMIOPort  Port=3  Side=Right
  Out- : PMIOPort  Port=4  Side=Right
  I : Outport
  V : Outport  Port=2
  wires:
  PS-Simulink Converter/1 -> I/1
  PS-Simulink Converter1/1 -> V/1
  connections:
  Voltage Sensor/LConn1 -- Current Sensor/RConn2 -- Out+/RConn1
  PS-Simulink Converter/LConn1 -- Current Sensor/RConn1
  Current Sensor/LConn1 -- In+/RConn1
  PS-Simulink Converter1/LConn1 -- Voltage Sensor/RConn1
  Voltage Sensor/RConn2 -- Out-/RConn1 -- In-/RConn1

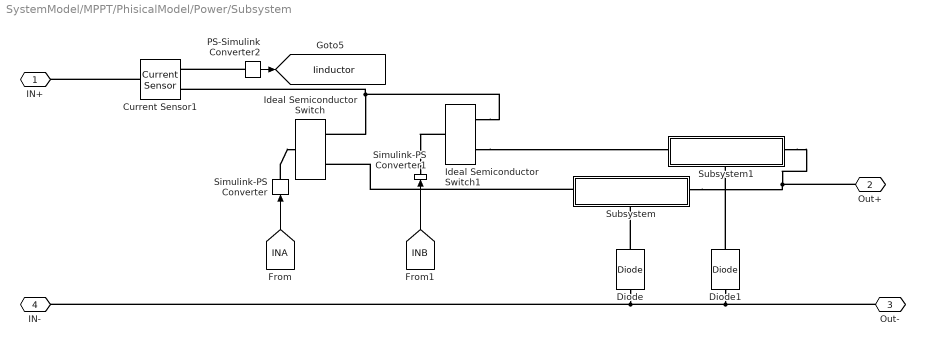
== system SystemModel/MPPT/PhisicalModel/Power/Subsystem ==
  Current Sensor1 : fl_lib/Electrical/Electrical Sensors/Current Sensor
  Diode : ee_lib/Semiconductors & Converters/Diode  ModelType=ee.enum.diode.modelType.pwl  IfMat=[.07, .12, .19, 1.75, 4.24, 7.32, 11.2; .16, .3, .72, 2.14, 4.02, 6.35, 9.12] A  TjVec=[25, 125] degC  VfVec=[.5, .7, .9, 1.3, 1.7, 2.1, 2.5] V  Vf=0.6 V  Ron=0.003 Ohm  Goff=1e-8 S  prmExp=ee.enum.diode.expParam.useTwo  I12=[.0137, .545] A  V12=[.6, .7] V  IS=1e-12 A  ec=1  I1=0.0137 A  V1=0.6 V  RS=0 Ohm  Tmeas=25 degC  N_series=1  N_parallel=1  Rz=0.3 Ohm  BV=inf V  C_param=ee.enum.diode.capParam.fixed  CJ=36 pF  CJ0=5 pF  VJ=1 V  Mgrad=0.5  Vvec=[.1, 10, 100] V  Cvec=[3.5, 1, .4] pF  FC=0.5  Q_param=ee.enum.diode.recoveryParam.off  iRM=-7.15 A  iF=4 A  didt=-750 A/us  trr_factor=3  trr=115 ns  Qrr=1500 s*uA  TT=50 ns  tau=100 ns  T_param=ee.enum.diode.temperatureParam.off  IS_T2=1.25e-7 A  I1_T2=0.245 A  V1_T2=0.5 V  Tmeas2=125 degC  EG_param=ee.enum.diode.egapParam.material_si  EG=1.11 eV  XTI_param=ee.enum.diode.xtiParam.pn  XTI=3  dBVdT=0 V/K  Tdevice=25 degC  i_specify=off  i_priority=None  i=0 A  i_nominal_specify=off  i_nominal_unit=A  i_nominal_value=1  v_specify=off  v_priority=None  v=0 V  v_nominal_specify=off  v_nominal_unit=V  v_nominal_value=1  i_capacitor_specify=off  i_capacitor_priority=None  i_capacitor=0 A  i_capacitor_nominal_specify=off  i_capacitor_nominal_unit=A  i_capacitor_nominal_value=1  v_capacitor_specify=off  v_capacitor_priority=None  v_capacitor=0 V  v_capacitor_nominal_specify=off  v_capacitor_nominal_unit=V  v_capacitor_nominal_value=1  power_dissipated_specify=off  power_dissipated_priority=None  power_dissipated=0 W  power_dissipated_nominal_specify=off  power_dissipated_nominal_unit=W  power_dissipated_nominal_value=1  thermal_network_parameterization=ee.enum.thermalNetworkTopology.cauer  Rth=[0, 10] K/W  Rth_Foster=[4, 6] K/W  thermal_mass_parameterization=ee.enum.thermalNetwork.timeconstant  thermal_mass=[0, 1] J/K  thermal_mass_Foster=[1.5, 3] J/K  thermal_time_constant=[0, 10] s  thermal_time_constant_Foster=[6, 18] s  thermal_mass_initial_temperatures=[25, 25] degC
  Diode1 : ee_lib/Semiconductors & Converters/Diode  ModelType=ee.enum.diode.modelType.pwl  IfMat=[.07, .12, .19, 1.75, 4.24, 7.32, 11.2; .16, .3, .72, 2.14, 4.02, 6.35, 9.12] A  TjVec=[25, 125] degC  VfVec=[.5, .7, .9, 1.3, 1.7, 2.1, 2.5] V  Vf=0.6 V  Ron=0.003 Ohm  Goff=1e-8 S  prmExp=ee.enum.diode.expParam.useTwo  I12=[.0137, .545] A  V12=[.6, .7] V  IS=1e-12 A  ec=1  I1=0.0137 A  V1=0.6 V  RS=0 Ohm  Tmeas=25 degC  N_series=1  N_parallel=1  Rz=0.3 Ohm  BV=inf V  C_param=ee.enum.diode.capParam.fixed  CJ=36 pF  CJ0=5 pF  VJ=1 V  Mgrad=0.5  Vvec=[.1, 10, 100] V  Cvec=[3.5, 1, .4] pF  FC=0.5  Q_param=ee.enum.diode.recoveryParam.off  iRM=-7.15 A  iF=4 A  didt=-750 A/us  trr_factor=3  trr=115 ns  Qrr=1500 s*uA  TT=50 ns  tau=100 ns  T_param=ee.enum.diode.temperatureParam.off  IS_T2=1.25e-7 A  I1_T2=0.245 A  V1_T2=0.5 V  Tmeas2=125 degC  EG_param=ee.enum.diode.egapParam.material_si  EG=1.11 eV  XTI_param=ee.enum.diode.xtiParam.pn  XTI=3  dBVdT=0 V/K  Tdevice=25 degC  i_specify=off  i_priority=None  i=0 A  i_nominal_specify=off  i_nominal_unit=A  i_nominal_value=1  v_specify=off  v_priority=None  v=0 V  v_nominal_specify=off  v_nominal_unit=V  v_nominal_value=1  i_capacitor_specify=off  i_capacitor_priority=None  i_capacitor=0 A  i_capacitor_nominal_specify=off  i_capacitor_nominal_unit=A  i_capacitor_nominal_value=1  v_capacitor_specify=off  v_capacitor_priority=None  v_capacitor=0 V  v_capacitor_nominal_specify=off  v_capacitor_nominal_unit=V  v_capacitor_nominal_value=1  power_dissipated_specify=off  power_dissipated_priority=None  power_dissipated=0 W  power_dissipated_nominal_specify=off  power_dissipated_nominal_unit=W  power_dissipated_nominal_value=1  thermal_network_parameterization=ee.enum.thermalNetworkTopology.cauer  Rth=[0, 10] K/W  Rth_Foster=[4, 6] K/W  thermal_mass_parameterization=ee.enum.thermalNetwork.timeconstant  thermal_mass=[0, 1] J/K  thermal_mass_Foster=[1.5, 3] J/K  thermal_time_constant=[0, 10] s  thermal_time_constant_Foster=[6, 18] s  thermal_mass_initial_temperatures=[25, 25] degC
  Ideal Semiconductor Switch : ee_lib/Semiconductors & Converters/Ideal Semiconductor Switch  Ron=0.001 Ohm  Goff=1e-6 1/Ohm  Vth=0.5 V  diode_param=2  diode_Vf=0.8 V  diode_Ron=0.001 Ohm  diode_Goff=1e-5 1/Ohm  diode_C=50e-9 F  diode_iRM=-235 A  diode_iF=300 A  diode_idot=-50 A/us  diode_trr_param=1  diode_trr_factor=3  diode_trr=15 us  diode_Qrr=1500 s*uA
      settings: SourceProductBaseCode=PS
  Ideal Semiconductor Switch1 : ee_lib/Semiconductors & Converters/Ideal Semiconductor Switch  Ron=0.001 Ohm  Goff=1e-6 1/Ohm  Vth=0.5 V  diode_param=2  diode_Vf=0.8 V  diode_Ron=0.001 Ohm  diode_Goff=1e-5 1/Ohm  diode_C=50e-9 F  diode_iRM=-235 A  diode_iF=300 A  diode_idot=-50 A/us  diode_trr_param=1  diode_trr_factor=3  diode_trr=15 us  diode_Qrr=1500 s*uA
      settings: SourceProductBaseCode=PS
  PS-Simulink Converter2 : nesl_utility/PS-Simulink Converter  PhysicalDomain=network_engine_domain  SubClassName=ps_output  LeftPortType=input  RightPortType=output  PseudoPeriodic=off  Frequencies=[]  Unit=inherit  AffineConversion=off
  Simulink-PS Converter : nesl_utility/Simulink-PS Converter  PhysicalDomain=network_engine_domain  SubClassName=ps_input  LeftPortType=input  RightPortType=output  PseudoPeriodic=off  Frequencies=[]  NoiseDistribution=none  NoiseParameters=[]  Unit=1  AffineConversion=off  FilteringAndDerivatives=provide  SimscapeFilterOrder=1  InputFilterTimeConstant=0.001  UdotUserProvided=0
  Simulink-PS Converter1 : nesl_utility/Simulink-PS Converter  PhysicalDomain=network_engine_domain  SubClassName=ps_input  LeftPortType=input  RightPortType=output  PseudoPeriodic=off  Frequencies=[]  NoiseDistribution=none  NoiseParameters=[]  Unit=1  AffineConversion=off  FilteringAndDerivatives=provide  SimscapeFilterOrder=1  InputFilterTimeConstant=0.001  UdotUserProvided=0
  Subsystem : Subsystem
      settings: PortSchema="{\"entries\":[{\"content\":{\"sides\":[{\"content\":{\"connectorIds\":[\"LConn1\"]},\"type\":\"ConnectorPlacement.EquallySpacedRectSide\",\"uuid\":\"64a96416-4874-4b36-bf76-485376ce2e10\"},{\"content\":{\"connectorIds\":[\"RConn1\"],\"side\":\"RIGHT\"},\"type\":\"ConnectorPlacement.EquallySpacedRectSide\",\"uuid\":\"55068a5e-3832-4911-967c-be8dd15c9dce\"},{\"content\":{\"connectorIds\":[],\"side\":\"TOP\"},\"type\":\"ConnectorPlacement.EquallySpacedRectSide\",\"uuid\":\"e6fe2f73-30be-404c-8b27-e0cd3feacb1a\"},{\"content\":{\"connectorIds\":[\"RConn2\"],\"side\":\"BOTTOM\"},\"type\":\"ConnectorPlacement.EquallySpacedRectSide\",\"uuid\":\"db9bece8-9e42-478a-b664-a23e99c2fe4f\"},{\"content\":{\"connectorIds\":[],\"side\":\"HIDDEN\"},\"type\":\"ConnectorPlacement.EquallySpacedRectSide\",\"uuid\":\"bd80cfeb-3a97-419b-bd5f-94c4a9539103\"}]},\"type\":\"ConnectorPlacement.EquallySpacedConnector\",\"uuid\":\"531a02a7-6f5c-4b11-87db-44817caedde7\"}],\"packageUris\":[\"http://schema.mathworks.com/mf0/Connector/R2020b\"],\"version\":\"1.0\"}"
  Subsystem1 : Subsystem
      settings: PortSchema="{\"entries\":[{\"content\":{\"sides\":[{\"content\":{\"connectorIds\":[\"LConn1\"]},\"type\":\"ConnectorPlacement.EquallySpacedRectSide\",\"uuid\":\"64a96416-4874-4b36-bf76-485376ce2e10\"},{\"content\":{\"connectorIds\":[\"RConn1\"],\"side\":\"RIGHT\"},\"type\":\"ConnectorPlacement.EquallySpacedRectSide\",\"uuid\":\"55068a5e-3832-4911-967c-be8dd15c9dce\"},{\"content\":{\"connectorIds\":[],\"side\":\"TOP\"},\"type\":\"ConnectorPlacement.EquallySpacedRectSide\",\"uuid\":\"e6fe2f73-30be-404c-8b27-e0cd3feacb1a\"},{\"content\":{\"connectorIds\":[\"RConn2\"],\"side\":\"BOTTOM\"},\"type\":\"ConnectorPlacement.EquallySpacedRectSide\",\"uuid\":\"db9bece8-9e42-478a-b664-a23e99c2fe4f\"},{\"content\":{\"connectorIds\":[],\"side\":\"HIDDEN\"},\"type\":\"ConnectorPlacement.EquallySpacedRectSide\",\"uuid\":\"bd80cfeb-3a97-419b-bd5f-94c4a9539103\"}]},\"type\":\"ConnectorPlacement.EquallySpacedConnector\",\"uuid\":\"531a02a7-6f5c-4b11-87db-44817caedde7\"}],\"packageUris\":[\"http://schema.mathworks.com/mf0/Connector/R2020b\"],\"version\":\"1.0\"}"
  IN+ : PMIOPort  Side=Left
  Out+ : PMIOPort  Port=2  Side=Right
  Out- : PMIOPort  Port=3  Side=Right
  IN- : PMIOPort  Port=4  Side=Left
  tag scope: Iinductor=global
  wires:
  [INB] -> Simulink-PS Converter1/1
  [INA] -> Simulink-PS Converter/1
  PS-Simulink Converter2/1 -> [Iinductor]
  connections:
  Simulink-PS Converter/RConn1 -- Ideal Semiconductor Switch/LConn1
  Ideal Semiconductor Switch1/RConn2 -- Subsystem1/LConn1
  Ideal Semiconductor Switch/RConn1 -- Current Sensor1/RConn2 -- Ideal Semiconductor Switch1/RConn1
  PS-Simulink Converter2/LConn1 -- Current Sensor1/RConn1
  Subsystem/LConn1 -- Ideal Semiconductor Switch/RConn2
  Ideal Semiconductor Switch1/LConn1 -- Simulink-PS Converter1/RConn1
  Current Sensor1/LConn1 -- IN+/RConn1
  Diode/LConn1 -- Diode1/LConn1 -- Out-/RConn1 -- IN-/RConn1
  Subsystem/RConn1 -- Subsystem1/RConn1 -- Out+/RConn1
  Diode/RConn1 -- Subsystem/RConn2
  Diode1/RConn1 -- Subsystem1/RConn2
